simulink model "steering"  (R2018b)
settings: Solver=VariableStepAuto  StartTime=0.0  StopTime=10  RelTol=1e-3
values from neighbouring files (symbols this model uses):
  D_steering_position = 0.0    (= 0)    [configuration.m]
  delay_tf_steering = 0    [configuration.m]
  den_tf_steering = [1 245.9 0]    [configuration.m]
  I_steering_position = 1    [configuration.m]    (also in simulate_bike.m = 30)
  K_feedforward_steering = 0    [configuration.m]
  num_tf_steering = [253.4]    [configuration.m]
  P_steering_position = 10    [configuration.m]    (also in simulate_bike.m = 30)
  Ts = 0.01    [configuration.m]    (also in configuration_pidTuning.m = 0.04)
undefined symbols (not defined in the file or in its folder): a_steering_filter, b_steering_filter
libraries: simulink_extras x3, simulink x1
settings Model: Creator=maximef  LastModifiedBy=maximef

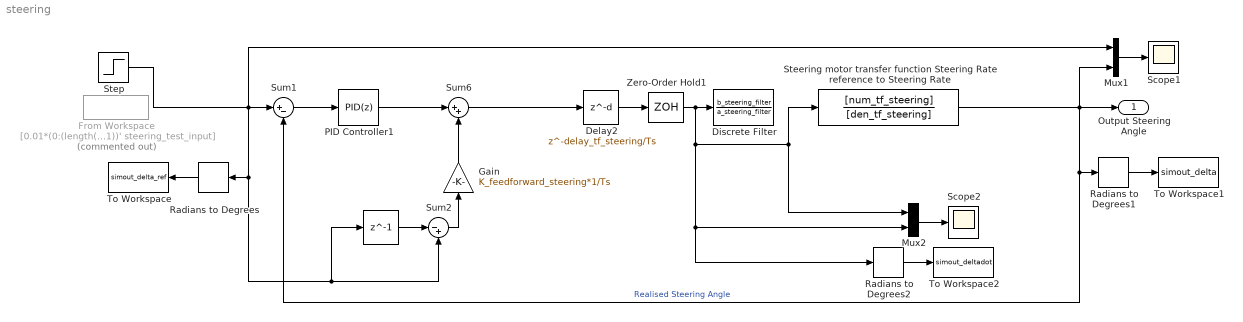
== system steering ==
  " " : Delay  DelayLength=1  SampleTime=Ts
  Delay2 : Delay  DelayLength=delay_tf_steering/Ts  SampleTime=Ts
  Discrete Filter : DiscreteFilter  Numerator=b_steering_filter  Denominator=a_steering_filter  SampleTime=Ts
  From Workspace : FromWorkspace  Commented=on  VariableName=[0.01*(0:(length(steering_test_input)-1))' steering_test_input]  SampleTime=0
  Gain : Gain  Gain=K_feedforward_steering*1/Ts
  Mux1 : Mux  Inputs=2
  Mux2 : Mux  Inputs=2
  PID Controller1 : simulink/Continuous/PID Controller  Controller=PID  Form=Parallel  TimeDomain=Discrete-time  SampleTime=Ts  IntegratorMethod=Forward Euler  FilterMethod=Forward Euler  ControllerParametersSource=internal  P=P_steering_position  I=I_steering_position  D=D_steering_position  UseFilter=off  N=1  TunerSelectOption=Transfer Function Based (PID Tuner App)  InitialConditionSource=internal  InitialConditionForIntegrator=0  InitialConditionForFilter=0  DifferentiatorICPrevScaledInput=0  ExternalReset=none  TrackingMode=off  Kt=1  LimitOutput=off  UpperSaturationLimit=inf  LowerSaturationLimit=-inf  LinearizeAsGain=on  AntiWindupMode=none  Kb=1  POutMin=[]  POutMax=[]  IOutMin=[]  IOutMax=[]  DOutMin=[]  DOutMax=[]  NOutMin=[]  NOutMax=[]  SumOutMin=[]  SumOutMax=[]  SaturationOutMin=[]  SaturationOutMax=[]  PParamMin=[]  PParamMax=[]  IParamMin=[]  IParamMax=[]  DParamMin=[]  DParamMax=[]  NParamMin=[]  NParamMax=[]  KbParamMin=[]  KbParamMax=[]  KtParamMin=[]  KtParamMax=[]  KbOutMin=[]  KbOutMax=[]  KtOutMin=[]  KtOutMax=[]  IntegratorOutMin=[]  IntegratorOutMax=[]  FilterOutMin=[]  FilterOutMax=[]  SumI1OutMin=[]  SumI1OutMax=[]  SumI2OutMin=[]  SumI2OutMax=[]  SumI3OutMin=[]  SumI3OutMax=[]  SumI4OutMin=[]  SumI4OutMax=[]  SumDOutMin=[]  SumDOutMax=[]  DifferentiatorOutMin=[]  DifferentiatorOutMax=[]  FilterDiffOutCoefMin=[]  FilterDiffOutCoefMax=[]  ReciprocalOutMin=[]  ReciprocalOutMax=[]  SumDenOutMin=[]  SumDenOutMax=[]  SumNumOutMin=[]  SumNumOutMax=[]  DivideOutMin=[]  DivideOutMax=[]  IntegratorContinuousStateAttributes=''  IntegratorStateMustResolveToSignalObject=off  IntegratorRTWStateStorageClass=Auto  FilterContinuousStateAttributes=''  FilterStateMustResolveToSignalObject=off  FilterRTWStateStorageClass=Auto  ParallelPVariant=InternalParameters  IdealPVariant=Disabled  IVariant=InternalParameters  DVariant=InternalParameters  IntegratorVariant=Discrete  SatVariant=Disabled  AWVariant=Passthrough  PCopyVariant=Disabled  TRVariant=Disabled  FdbkBlocksVariant=Forward  IdealPFdbkVariant=Disabled  SatFdbkVariant=Disabled  DerivativeFilterVariant=Differentiator  NVariant=Passthrough  NCopyVariant=Disabled_SignalSpec  FilterICVariant=InternalICsDifferentiator  IntegratorICVariant=InternalICs  ExternalResetVariant=Disabled  TRSumVariant=Passthrough  SumFdbkVariant=Disabled  SumVariant=Sum_PID
  Radians to Degrees : simulink_extras/Transformations/Radians to Degrees
  Radians to Degrees1 : simulink_extras/Transformations/Radians to Degrees
  Radians to Degrees2 : simulink_extras/Transformations/Radians to Degrees
  Scope1 : Scope
  Scope2 : Scope
  Steering motor transfer function Steering Rate reference to Steering Rate : TransferFcn  Numerator=[num_tf_steering]  Denominator=[den_tf_steering]
  Step : Step  Time=0  After=deg2rad(5)  SampleTime=0
  Sum1 : Sum  Inputs=|+-
  Sum2 : Sum  Inputs=|-+
  Sum6 : Sum  Inputs=|++
  To Workspace : ToWorkspace  VariableName=simout_delta_ref  SaveFormat=Timeseries  SampleTime=-1
  To Workspace1 : ToWorkspace  VariableName=simout_delta  SaveFormat=Timeseries  SampleTime=-1
  To Workspace2 : ToWorkspace  VariableName=simout_deltadot  SaveFormat=Timeseries  SampleTime=-1
  Zero-Order Hold1 : ZeroOrderHold  SampleTime=Ts
  Output Steering Angle : Outport
  wires:
  Steering motor transfer function Steering Rate reference to Steering Rate/1 -> Mux1/2, Radians to Degrees1/1, Sum1/2, Output Steering Angle/1  "Realised Steering Angle"
  Zero-Order Hold1/1 -> Steering motor transfer function Steering Rate reference to Steering Rate/1, Mux2/1, Radians to Degrees2/1, Mux2/2, Discrete Filter/1
  Mux2/1 -> Scope2/1
  Sum2/1 -> Gain/1
  Sum1/1 -> PID Controller1/1
  Sum6/1 -> Delay2/1
  " "/1 -> Sum2/1
  Mux1/1 -> Scope1/1
  Step/1 -> Mux1/1, Radians to Degrees/1, Sum2/2, " "/1, Sum1/1
  Delay2/1 -> Zero-Order Hold1/1
  Radians to Degrees/1 -> To Workspace/1
  Radians to Degrees1/1 -> To Workspace1/1
  PID Controller1/1 -> Sum6/1
  Radians to Degrees2/1 -> To Workspace2/1
  Gain/1 -> Sum6/2
